simulink model "FBRModel"  (R2021a)
settings: Solver=VariableStepAuto  StartTime=0.0  StopTime=2  FixedStep=0.01  RelTol=1e-3
PreLoadFcn:
  | TP_TASK_SPACE = Simulink.Variant('TP_MODE==1');
  | TP_JOINT_SPACE = Simulink.Variant('TP_MODE==2');
InitFcn:
  | if TP_MODE == 1
  |     %pass
  |     return;
  | end
  | jointWaypoints = zeros(4, size(waypoints, 2));
  | for i=1:size(waypoints, 2)
  |     config = FBR.searchConfiguration( ...
  |         FBR.solveIK(bodyLengths.La, bodyLengths.Lb, bodyLengths.Lc, waypoints(1, i), waypoints(2, i)) ...
  |     );
  |     jointWaypoints(:, i) = [config.th1; config.th2; config.th3; config.th4];
  | end
undefined symbols (not defined in the file): bodyLengths, waypoints, waypointTimes
libraries: robotcorelib x2
settings Model: Creator=chiar  LastModifiedBy=chiar
settings OptimizationCC: BlockReduction=off  DefaultParameterBehavior=Inlined  BufferReuse=off

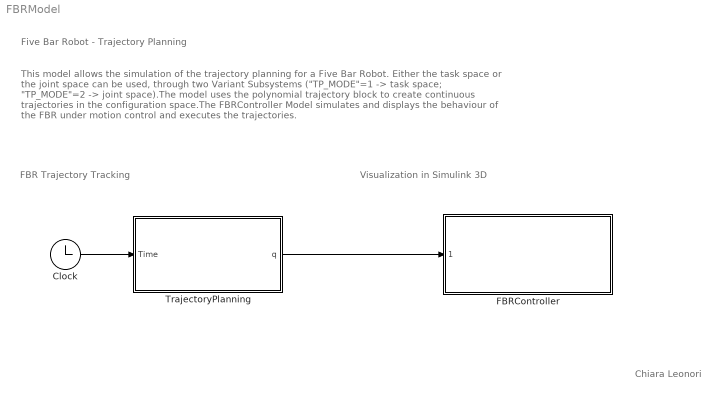
== system FBRModel ==
  note: Chiara Leonori
  note: FBR Trajectory Tracking
  note: Visualization in Simulink 3D
  note: This model allows the simulation of the trajectory planning for a Five Bar Robot. Either the task space or the joint space can be used, through two Variant Subsystems ("TP_MODE"=1 -> task space; "TP_MODE"=2 -> joint space).The model uses the polynomial trajectory block to create continuous trajectories in the configuration space.The FBRController Model simulates and displays the behaviour of the FBR under motion control and executes the trajectories.
  note: Five Bar Robot - Trajectory Planning
  Clock : Clock
  FBRController : Subsystem  ReferencedSubsystem=FBRController
  TrajectoryPlanning : Subsystem  Variant=on
  wires:
  TrajectoryPlanning/1(q) -> FBRController/1
  Clock/1 -> TrajectoryPlanning/1(Time)

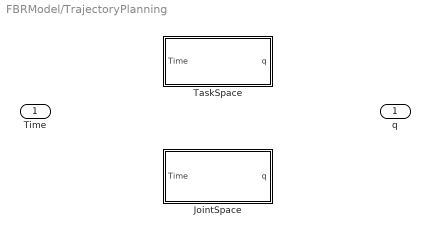
== system FBRModel/TrajectoryPlanning ==
  Time : Inport
  JointSpace : Subsystem  VariantControl=TP_MODE == 2
  TaskSpace : Subsystem  VariantControl=TP_MODE == 1
  q : Outport  OutDataTypeStr=Bus: Bus_q

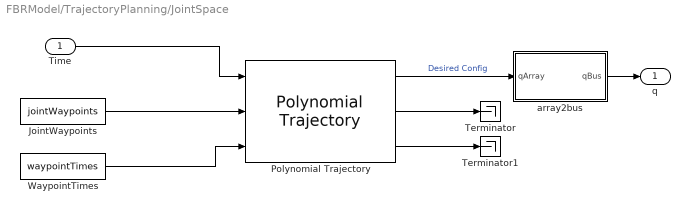
== system FBRModel/TrajectoryPlanning/JointSpace ==
  Time : Inport
  JointWaypoints : Constant  Value=jointWaypoints
  Polynomial Trajectory : robotcorelib/Polynomial Trajectory  WaypointSource=External  TimePoints=[ 0, 1, 2, 3, 4 ]  TimeInterval=[ 1, 4 ]  Method=Cubic Polynomial  ParameterSource=Internal  VelocityBoundaryCondition=zeros( 4, size(waypoints, 2) )  AccelerationBoundaryCondition=zeros( 2, 5 )  SimulateUsing=Interpreted execution
  Terminator : Terminator
  Terminator1 : Terminator
  WaypointTimes : Constant  Value=waypointTimes
  array2bus : MATLAB Function  TreatAsAtomicUnit=on
  q : Outport  OutDataTypeStr=Bus: Bus_q
  wires:
  Time/1 -> Polynomial Trajectory/1
  Polynomial Trajectory/2 -> Terminator/1
  Polynomial Trajectory/3 -> Terminator1/1
  WaypointTimes/1 -> Polynomial Trajectory/3
  Polynomial Trajectory/1 -> array2bus/1(qArray)  "Desired Config"
  array2bus/1(qBus) -> q/1
  JointWaypoints/1 -> Polynomial Trajectory/2

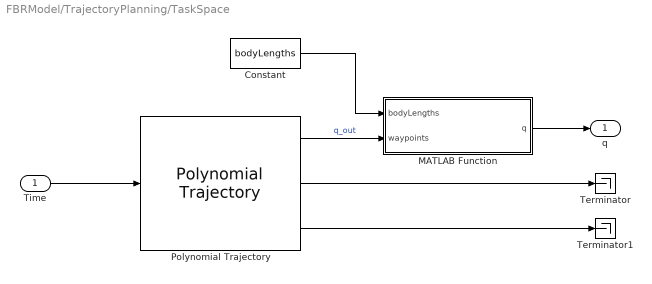
== system FBRModel/TrajectoryPlanning/TaskSpace ==
  Time : Inport
  Constant : Constant  Value=bodyLengths  OutDataTypeStr=Bus: Bus_BodyLengths
  MATLAB Function : MATLAB Function  TreatAsAtomicUnit=on
  Polynomial Trajectory : robotcorelib/Polynomial Trajectory  WaypointSource=Internal  Waypoints=waypoints  TimePoints=waypointTimes  TimeInterval=[ 1, 4 ]  Method=Cubic Polynomial  ParameterSource=Internal  VelocityBoundaryCondition=waypointVels  AccelerationBoundaryCondition=zeros( 2, 5 )  SimulateUsing=Interpreted execution
  Terminator : Terminator
  Terminator1 : Terminator
  q : Outport  OutDataTypeStr=Bus: Bus_q
  wires:
  Time/1 -> Polynomial Trajectory/1
  Polynomial Trajectory/2 -> Terminator/1
  Polynomial Trajectory/3 -> Terminator1/1
  Constant/1 -> MATLAB Function/1(bodyLengths)
  Polynomial Trajectory/1 -> MATLAB Function/2(waypoints)  "q_out"
  MATLAB Function/1(q) -> q/1

== matlab function FBRModel/TrajectoryPlanning/JointSpace/array2bus ==
  data: qArray input; qBus output Bus: Bus_q
function qBus = adapter(qArray)
    qBus.th1 = qArray(1);
    qBus.th2 = qArray(2);
    qBus.th3 = qArray(3);
    qBus.th4 = qArray(4);

== matlab function FBRModel/TrajectoryPlanning/TaskSpace/MATLAB Function ==
  data: bodyLengths input Bus: Bus_BodyLengths; q output Bus: Bus_q; waypoints input
function q = IKSolver(bodyLengths, waypoints)

solution = FBR.solveIK(bodyLengths.La, bodyLengths.Lb, bodyLengths.Lc, waypoints(1), waypoints(2));
qComplete = FBR.searchConfiguration(solution);
q.th1 = qComplete.th1;
q.th2 = qComplete.th2;
q.th3 = qComplete.th3;
q.th4 = qComplete.th4;
